simulink model "TestingObs"  (R2019b)
settings: Solver=VariableStepAuto  StartTime=0.0  StopTime=10.0  RelTol=1e-3
settings Model: Creator=shahidyaqoob  LastModifiedBy=aarij
settings DataIOCC: ReturnWorkspaceOutputs=off
settings DebuggingCC: ArithmeticOperatorsInVariantConditions=warning
settings SFSimCC: CustomCodeUndefinedFunction=UseInterfaceOnly

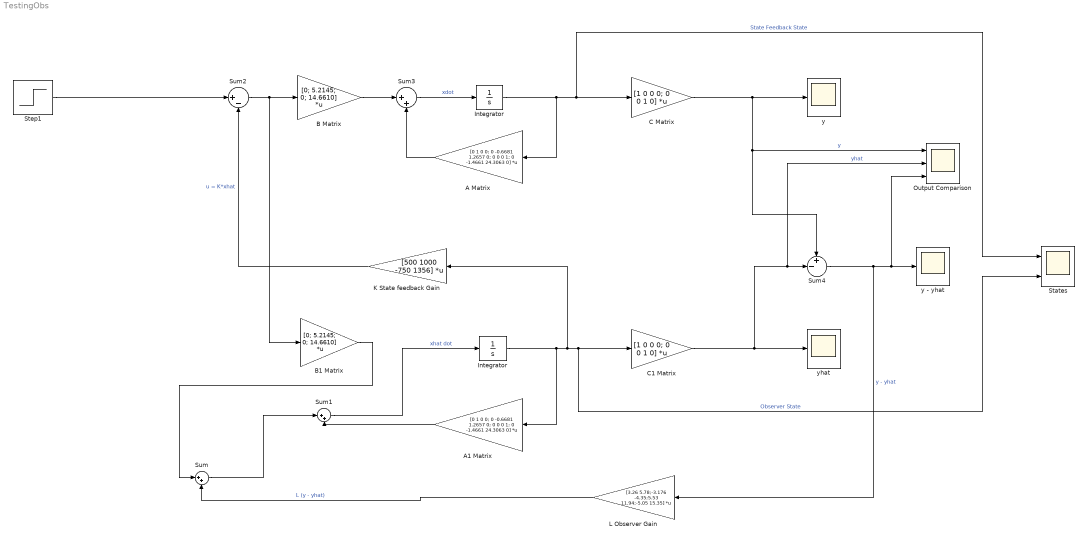
== system TestingObs ==
  A Matrix : Gain  Gain=[0 1 0 0; 0 -0.6681 1.2657 0; 0 0 0 1; 0 -1.4661 24.3063 0]  Multiplication=Matrix(K*u)
  A1 Matrix : Gain  Gain=[0 1 0 0; 0 -0.6681 1.2657 0; 0 0 0 1; 0 -1.4661 24.3063 0]  Multiplication=Matrix(K*u)
  B Matrix : Gain  Gain=[0; 5.2145; 0; 14.6610]  Multiplication=Matrix(K*u) (u vector)
  B1 Matrix : Gain  Gain=[0; 5.2145; 0; 14.6610]  Multiplication=Matrix(K*u)
  C Matrix : Gain  Gain=[1 0 0 0; 0 0 1 0]  Multiplication=Matrix(K*u) (u vector)
  C1 Matrix : Gain  Gain=[1 0 0 0; 0 0 1 0]  Multiplication=Matrix(K*u)
  "Integrator " : Integrator  InitialCondition=[0 0 0 0]
  "Integrator " : Integrator  InitialCondition=[0 0 0 0]
  K State feedback Gain : Gain  Gain=[500 1000 -750 1356]  Multiplication=Matrix(K*u) (u vector)
  L Observer Gain : Gain  Gain=[3.26 5.78;-3.176 -4.35;5.53 11.94;-5.05 15.35]  Multiplication=Matrix(K*u) (u vector)
  Output Comparison : Scope  NumInputPorts=3
  States : Scope  NumInputPorts=2
  Step1 : Step  Time=0  SampleTime=0
  Sum : Sum  Inputs=|++
  Sum1 : Sum  Inputs=|++
  Sum2 : Sum  Inputs=|+-
  Sum3 : Sum  Inputs=|++
  Sum4 : Sum  Inputs=+-|
  y : Scope
  y - yhat : Scope
  yhat : Scope
  wires:
  K State feedback Gain/1 -> Sum2/2  "u = K*xhat"
  Sum1/1 -> "Integrator "/1  "xhat dot"
  A Matrix/1 -> Sum3/2
  C Matrix/1 -> Output Comparison/1, Sum4/1, y/1  "y"
  "Integrator "/1 -> C1 Matrix/1, States/2, K State feedback Gain/1, A1 Matrix/1  "Observer State"
  B Matrix/1 -> Sum3/1
  Sum3/1 -> "Integrator "/1  "xdot"
  "Integrator "/1 -> A Matrix/1, C Matrix/1, States/1  "State Feedback State"
  Sum2/1 -> B Matrix/1, B1 Matrix/1
  B1 Matrix/1 -> Sum/1
  L Observer Gain/1 -> Sum/2  "L (y - yhat)"
  C1 Matrix/1 -> yhat/1, Output Comparison/2, Sum4/2  "yhat"
  Sum4/1 -> Output Comparison/3, y - yhat/1, L Observer Gain/1  "y - yhat"
  A1 Matrix/1 -> Sum1/2
  Step1/1 -> Sum2/1
  Sum/1 -> Sum1/1
